simulink model "MS_Mesure_Rs"  (R2021b)
settings: Solver=ode45  StartTime=0.0  StopTime=2  MaxStep=100e-6  RelTol=1e-6  EnableMultiTasking=on
undefined symbols (not defined in the file): Ts
libraries: powerlib_extras x3, spsControlledVoltageSourceLib x1, spsGroundLib x1, spsPermanentMagnetSynchronousMachineLib x1, spspowerguiLib x1
settings Model: Creator=obethoux  LastModifiedBy=zhifansong
settings SolverCC: AlgebraicLoopSolver=TrustRegion
settings DataIOCC: LimitDataPoints=on  SaveFormat=Array  SignalLoggingSaveFormat=ModelDataLogs  ReturnWorkspaceOutputs=off
settings OptimizationCC: ExpressionDepthLimit=2147483647  LifeSpan=inf
settings DebuggingCC: UnderspecifiedInitializationDetection=Classic  MergeDetectMultiDrivingBlocksExec=none  SolverPrmCheckMsg=warning  FcnCallInpInsideContextMsg=warning  StateNameClashWarn=warning  SFUnexpectedBacktrackingDiag=warning  SFNoUnconditionalDefaultTransitionDiag=warning  SFExecutionAtInitializationDiag=none  SFMachineParentedDataDiag=warning  ArithmeticOperatorsInVariantConditions=warning
settings HardwareCC: ProdBitPerPointer=32  ProdBitPerSizeT=32  ProdBitPerPtrDiffT=32  ProdLargestAtomicFloat=None  ProdIntDivRoundTo=Undefined  ProdEndianess=Unspecified  ProdWordSize=32  ProdHWDeviceType=32-bit Generic
settings ModelReferenceCC: PropagateSignalLabelsOutOfModel=off
settings SFSimCC: SimUseLocalCustomCode=off  CustomCodeUndefinedFunction=UseInterfaceOnly
settings RTWCC: RTWUseLocalCustomCode=off
settings CodeAppCC: StateflowObjectComments=on
settings GRTTargetCC: TargetLangStandard=C89/C90 (ANSI)  CombineOutputUpdateFcns=off  GRTInterface=on
settings ConfigComp: CovMetricSettings=dw  CovSaveCumulativeToWorkspaceVar=on  CovSaveSingleToWorkspaceVar=on  CovExternalEMLEnable=off
settings SimscapeCC: SimscapeNormalizeSystem=off

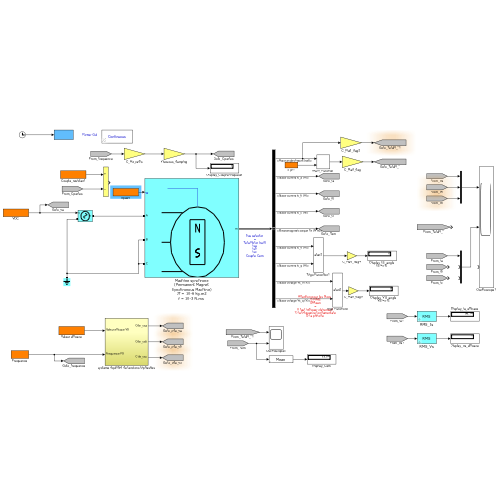
[thumbnail: Simulink's stored preview of the top-level diagram]
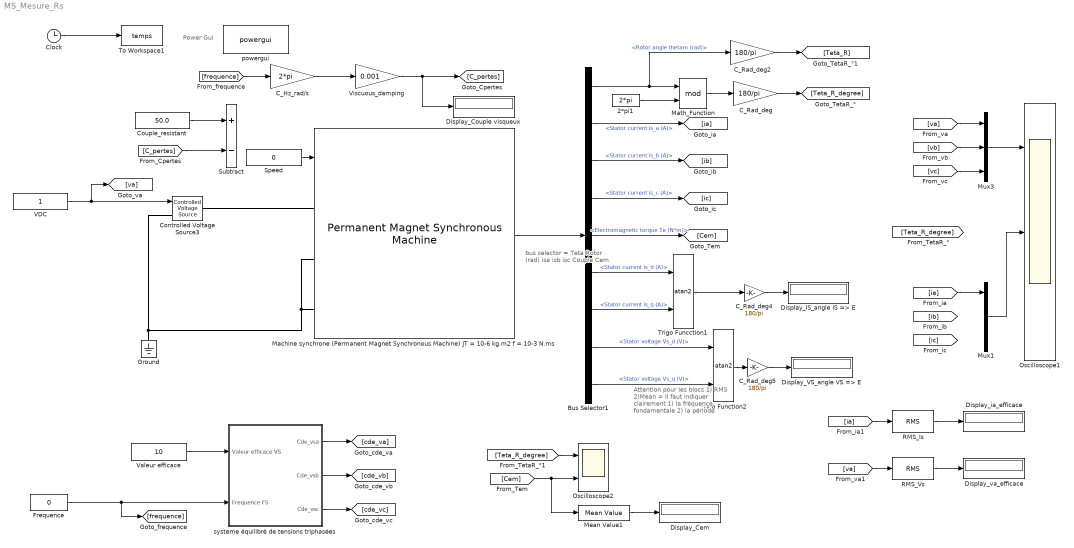
== system MS_Mesure_Rs ==
  note: Power Gui
  note: bus selector
      | =
      | Teta Rotor (rad)
      | isa
      | isb
      | isc
      | Couple Cem
  note: Attention pour les blocs
      | 1) RMS
      | 2)Mean
      | =
      | Il faut indiquer clairement
      | 1) la fréquence fondamentale
      | 2) la période
  2*pi1 : Constant  Value=2*pi
  Bus Selector1 : BusSelector  OutputSignals=Rotor angle thetam (rad),Stator current is_a (A),Stator current is_b (A),Stator current is_c (A),Electromagnetic torque Te (N*m),Stator current is_d (A),Stator current is_q (A),Stator voltage Vs_d (V),Stator voltage Vs_q (V)
  C_Hz_rad/s : Gain  Gain=2*pi
  C_Rad_deg{,2,4..5} (4 alike) : Gain  Gain=180/pi
  Clock : Clock
  Controlled Voltage Source3 : spsControlledVoltageSourceLib/Controlled Voltage Source  Initialize=on  Source_Type=DC  Amplitude=0  Phase=0  Frequency=0  Measurements=None
  Couple_resistant : Constant  Value=50.0
  Display_Cem : Display
  Display_Couple visqueux : Display
      settings: Decimation=100
  Display_IS_angle IS => E : Display
      settings: Decimation=100
  Display_VS_angle VS => E : Display
      settings: Decimation=100
  Display_ia_efficace : Display
  Display_va_efficace : Display
  Frequence : Constant  Value=0
  Ground : spsGroundLib/Ground  LConnTagsString=a
  "Machine synchrone (Permanent Magnet Synchronous Machine) JT = 10-6 kg.m2 f = 10-3 N.ms " : spsPermanentMagnetSynchronousMachineLib/Permanent Magnet Synchronous Machine  NbPhases=3  FluxDistribution=Sinusoidal  RotorType=Round  MechanicalLoad=Speed w  PresetModel=No  ShowDetailedParameters=on  MeasurementBus=off  Resistance=6.75e-3  Inductance=8.5e-3  dqInductances=[8.5e-3,8.5e-3]  La=1.61e-3  MachineConstant=Flux linkage established by magnets (V.s)  Flux=358.1e-3  VoltageCst=64.9522  TorqueCst=0.53715  Flat=120  Mechanical=[1e-6 1e-3 1 0]  PolePairs=1  InitialConditions=[0,0, 0,0]  InitialConditions5ph=[0 0 0 0 0 0]  RefAngle=90 degrees behind phase A axis (modified Park)  IterativeDiscreteModel=Trapezoidal non iterative  TsBlock=-1  TsPowergui=0
  Math_Function : Math  Operator=mod  SignedPower=on  SaturateOnIntegerOverflow=on
  Mean Value1 : powerlib_extras/Measurements/Mean Value  Period=inv(100)
      settings: SourceProductBaseCode=PS
  Mux1 : Mux  Inputs=3
  Mux3 : Mux  Inputs=3
  Oscilloscope1 : Scope  NumInputPorts=3
  Oscilloscope2 : Scope  NumInputPorts=2
  RMS_Is : powerlib_extras/Measurements/RMS  f1=100
      settings: SourceProductBaseCode=PS
  RMS_Vs : powerlib_extras/Measurements/RMS  f1=100
      settings: SourceProductBaseCode=PS
  Speed : Constant  Value=0
  Subtract : Sum  Inputs=+-
  To Workspace1 : ToWorkspace  VariableName=temps  SampleTime=-1
  Trigo Funcction1 : Trigonometry  Operator=atan2
  Trigo Function2 : Trigonometry  Operator=atan2
  VDC : Constant
  Valeur efficace : Constant  Value=10
  Viscuous_damping : Gain  Gain=0.001
  powergui : spspowerguiLib/powergui  Priority=2  SimulationMode=Continuous  SampleTime=Ts  frequency=60  Iterations=50  frequencyindice=0  Pbase=100e6  ErrMax=1e-4  UnitsV=kV  UnitsW=MW  buscounter=0  FunctionMessages=off  echomessages=off  EnableUseOfTLC=off  CurrentSourceSwitches=off  DisableSnubberDevices=off  DisableRonSwitches=off  DisableVfSwitches=off  DisplayEquations=off  AutomaticDiscreteSolvers=off  SolverType=Tustin  Interpol=off  ExternalGateDelay=off  methode=off  Ts=0  x0status=blocks  SPID=off  SwTol=0  HookPort=off  NonlinearTolerance=1e-4  nMaxIteration=100  ContinueOnMaxIteration=off  RestoreLinks=warning  ResistiveCurrentMeasurement=off  Frange=[0:2:500]  Ylog=off  Xlog=on  ShowGrid=off  save=off  variable=ZData  structure=0  ZoomFFT=on  StartTime=0.0  cycles=1  DisplayStyle=1  fundamental=60  FreqAxis=off  MaxFrequency=1000  frequencyindicesteady=1  RmsSteady=1  display=off
  systeme équilibré de tensions triphasées : Subsystem
  wires:
  Clock/1 -> To Workspace1/1
  "Machine synchrone (Permanent Magnet Synchronous Machine) JT = 10-6 kg.m2 f = 10-3 N.ms "/1 -> Bus Selector1/1
  Mux3/1 -> Oscilloscope1/1
  [ia] -> Mux1/1
  [va] -> Mux3/1
  [vb] -> Mux3/2
  [vc] -> Mux3/3
  Valeur efficace/1 -> systeme équilibré de tensions triphasées/1(Valeur efficace VS)
  Frequence/1 -> systeme équilibré de tensions triphasées/2(Frequence FS), [frequence]
  systeme équilibré de tensions triphasées/1(Cde_vsa) -> [cde_va]
  systeme équilibré de tensions triphasées/2(Cde_vsb) -> [cde_vb]
  systeme équilibré de tensions triphasées/3(Cde_vsc) -> [cde_vc]
  VDC/1 -> Controlled Voltage Source3/1, [va]
  [ia] -> RMS_Is/1
  RMS_Is/1 -> Display_ia_efficace/1
  [va] -> RMS_Vs/1
  RMS_Vs/1 -> Display_va_efficace/1
  [Teta_R_degree] -> Oscilloscope2/1
  [Cem] -> Oscilloscope2/2, Mean Value1/1
  [frequence] -> C_Hz_rad/s/1
  C_Hz_rad/s/1 -> Viscuous_damping/1
  Viscuous_damping/1 -> [C_pertes], Display_Couple visqueux/1
  Mean Value1/1 -> Display_Cem/1
  Couple_resistant/1 -> Subtract/1
  [C_pertes] -> Subtract/2
  Bus Selector1/1 -> Math_Function/1, C_Rad_deg2/1  "<Rotor angle thetam (rad)>"
  2*pi1/1 -> Math_Function/2
  Math_Function/1 -> C_Rad_deg/1
  Bus Selector1/2 -> [ia]  "<Stator current is_a (A)>"
  Bus Selector1/3 -> [ib]  "<Stator current is_b (A)>"
  Bus Selector1/4 -> [ic]  "<Stator current is_c (A)>"
  Bus Selector1/5 -> [Cem]  "<Electromagnetic torque Te (N*m)>"
  C_Rad_deg/1 -> [Teta_R_degree]
  C_Rad_deg2/1 -> [Teta_R]
  Trigo Funcction1/1 -> C_Rad_deg4/1
  Trigo Function2/1 -> C_Rad_deg5/1
  C_Rad_deg4/1 -> Display_IS_angle IS => E/1
  C_Rad_deg5/1 -> Display_VS_angle VS => E/1
  Bus Selector1/6 -> Trigo Funcction1/1  "<Stator current is_d (A)>"
  Bus Selector1/7 -> Trigo Funcction1/2  "<Stator current is_q (A)>"
  Bus Selector1/8 -> Trigo Function2/1  "<Stator voltage Vs_d (V)>"
  Bus Selector1/9 -> Trigo Function2/2  "<Stator voltage Vs_q (V)>"
  Speed/1 -> "Machine synchrone (Permanent Magnet Synchronous Machine) JT = 10-6 kg.m2 f = 10-3 N.ms "/1
  Mux1/1 -> Oscilloscope1/2
  connections:
  "Machine synchrone (Permanent Magnet Synchronous Machine) JT = 10-6 kg.m2 f = 10-3 N.ms "/LConn2 -- Controlled Voltage Source3/LConn1 -- Ground/LConn1 -- "Machine synchrone (Permanent Magnet Synchronous Machine) JT = 10-6 kg.m2 f = 10-3 N.ms "/LConn3
  "Machine synchrone (Permanent Magnet Synchronous Machine) JT = 10-6 kg.m2 f = 10-3 N.ms "/LConn1 -- Controlled Voltage Source3/RConn1

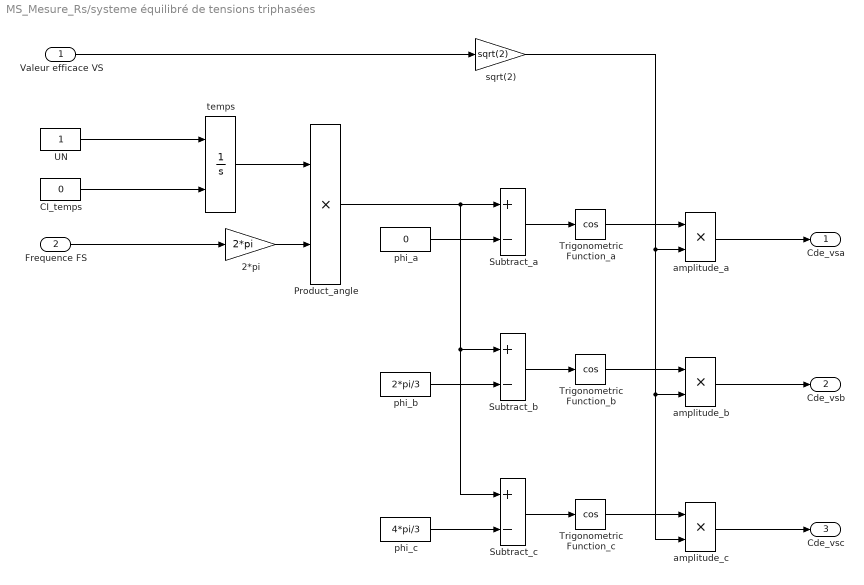
== system MS_Mesure_Rs/systeme équilibré de tensions triphasées ==
  Valeur efficace VS : Inport
  Frequence FS : Inport  Port=2
  2*pi : Gain  Gain=2*pi
  CI_temps : Constant  Value=0
  Product_angle : Product  RndMeth=Zero
  Subtract_a : Sum  Inputs=+-
  Subtract_b : Sum  Inputs=+-
  Subtract_c : Sum  Inputs=+-
  Trigonometric Function_a : Trigonometry  Operator=cos
  Trigonometric Function_b : Trigonometry  Operator=cos
  Trigonometric Function_c : Trigonometry  Operator=cos
  UN : Constant
  amplitude_a : Product  RndMeth=Zero
  amplitude_b : Product  RndMeth=Zero
  amplitude_c : Product  RndMeth=Zero
  phi_a : Constant  Value=0
  phi_b : Constant  Value=2*pi/3
  phi_c : Constant  Value=4*pi/3
  sqrt(2) : Gain  Gain=sqrt(2)
  temps : Integrator  InitialConditionSource=external
  Cde_vsa : Outport
  Cde_vsb : Outport  Port=2
  Cde_vsc : Outport  Port=3
  wires:
  CI_temps/1 -> temps/2
  UN/1 -> temps/1
  temps/1 -> Product_angle/1
  2*pi/1 -> Product_angle/2
  Product_angle/1 -> Subtract_a/1, Subtract_b/1, Subtract_c/1
  phi_a/1 -> Subtract_a/2
  phi_b/1 -> Subtract_b/2
  phi_c/1 -> Subtract_c/2
  Subtract_a/1 -> Trigonometric Function_a/1
  Subtract_b/1 -> Trigonometric Function_b/1
  Subtract_c/1 -> Trigonometric Function_c/1
  Trigonometric Function_a/1 -> amplitude_a/1
  Trigonometric Function_b/1 -> amplitude_b/1
  Trigonometric Function_c/1 -> amplitude_c/1
  sqrt(2)/1 -> amplitude_a/2, amplitude_b/2, amplitude_c/2
  Valeur efficace VS/1 -> sqrt(2)/1
  amplitude_a/1 -> Cde_vsa/1
  Frequence FS/1 -> 2*pi/1
  amplitude_b/1 -> Cde_vsb/1
  amplitude_c/1 -> Cde_vsc/1
